simulink model "GolfSwing3D_SimscapePhysicalInterfaceSwitching"  (R2024b)
settings: Solver=VariableStepAuto  StartTime=0.0  StopTime=StopTime  MaxStep=0.001  RelTol=1e-3
model workspace: external: MAT-File 3DModelInputs.mat (data not in the file)
undefined symbols (not defined in the file): GripStrength, KillswitchFinalValue, KillswitchInitialValue, KillswitchStepTime, LeftLowerArmLength, PlaneTilt, RightLowerArmLength, UpperTorsoLength, X, Y, Z
libraries: nesl_utility x363, sm_lib x137, matrix_library x11, fl_lib x8, simulink x1
(part 5 of 13)

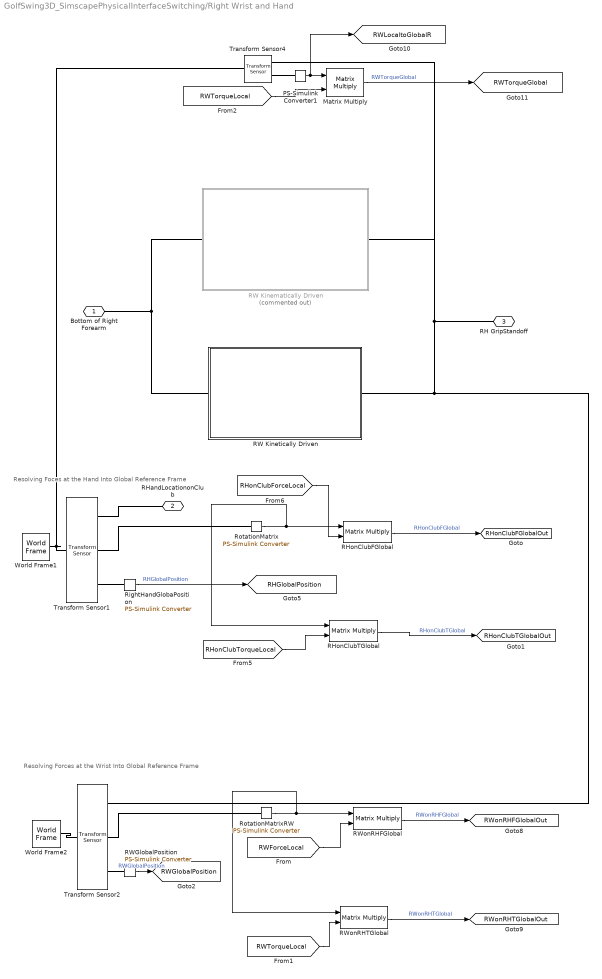
== system GolfSwing3D_SimscapePhysicalInterfaceSwitching/Right Wrist and Hand ==
  note: Resolving Foces at the Hand Into Global Reference Frame
  note: Resolving Forces at the Wrist Into Global Reference Frame
  Matrix Multiply : Product  Multiplication=Matrix(*)
  PS-Simulink Converter1 : nesl_utility/PS-Simulink Converter  PhysicalDomain=network_engine_domain  SubClassName=ps_output  LeftPortType=input  RightPortType=output  PseudoPeriodic=off  Frequencies=[]  VectorFormat=1-D array  Unit=inherit  AffineConversion=off
  RHonClubFGlobal : Product  Multiplication=Matrix(*)
  RHonClubTGlobal : Product  Multiplication=Matrix(*)
  RW Kinematically Driven : Subsystem  Commented=on
  RW Kinetically Driven : Subsystem
  RWGlobalPosition : nesl_utility/PS-Simulink Converter  PhysicalDomain=network_engine_domain  SubClassName=ps_output  LeftPortType=input  RightPortType=output  PseudoPeriodic=off  Frequencies=[]  VectorFormat=1-D array  Unit=inherit  AffineConversion=off
  RWonRHFGlobal : Product  Multiplication=Matrix(*)
  RWonRHTGlobal : Product  Multiplication=Matrix(*)
  RightHandGlobaPosition : nesl_utility/PS-Simulink Converter  PhysicalDomain=network_engine_domain  SubClassName=ps_output  LeftPortType=input  RightPortType=output  PseudoPeriodic=off  Frequencies=[]  VectorFormat=1-D array  Unit=inherit  AffineConversion=off
  RotationMatrix : nesl_utility/PS-Simulink Converter  PhysicalDomain=network_engine_domain  SubClassName=ps_output  LeftPortType=input  RightPortType=output  PseudoPeriodic=off  Frequencies=[]  VectorFormat=1-D array  Unit=inherit  AffineConversion=off
  RotationMatrixRW : nesl_utility/PS-Simulink Converter  PhysicalDomain=network_engine_domain  SubClassName=ps_output  LeftPortType=input  RightPortType=output  PseudoPeriodic=off  Frequencies=[]  VectorFormat=1-D array  Unit=inherit  AffineConversion=off
  Transform Sensor1 : sm_lib/Frames and Transforms/Transform Sensor  MeasurementFrame=World  RotationSequence=XYX  SenseAngle=off  SenseAxis=off  SenseQ=off  SenseR=on  SenseRotationSequence=off  SenseOmegaX=off  SenseOmegaY=off  SenseOmegaZ=off  SenseOmega=off  SenseQDot=off  SenseRDot=off  SenseRotationSequenceDot=off  SenseAlphaX=off  SenseAlphaY=off  SenseAlphaZ=off  SenseAlpha=off  SenseQDDot=off  SenseRDDot=off  SenseX=off  SenseY=off  SenseZ=off  SenseXYZ=on  SenseRad=off  SenseAzim=off  SenseDist=off  SenseInc=off  SenseXDot=off  SenseYDot=off  SenseZDot=off  SenseXYZDot=off  SenseRadDot=off  SenseAzimDot=off  SenseDistDot=off  SenseIncDot=off  SenseXDDot=off  SenseYDDot=off  SenseZDDot=off  SenseXYZDDot=off  SenseRadDDot=off  SenseAzimDDot=off  SenseDistDDot=off  SenseIncDDot=off
  Transform Sensor2 : sm_lib/Frames and Transforms/Transform Sensor  MeasurementFrame=World  RotationSequence=XYX  SenseAngle=off  SenseAxis=off  SenseQ=off  SenseR=on  SenseRotationSequence=off  SenseOmegaX=off  SenseOmegaY=off  SenseOmegaZ=off  SenseOmega=off  SenseQDot=off  SenseRDot=off  SenseRotationSequenceDot=off  SenseAlphaX=off  SenseAlphaY=off  SenseAlphaZ=off  SenseAlpha=off  SenseQDDot=off  SenseRDDot=off  SenseX=off  SenseY=off  SenseZ=off  SenseXYZ=on  SenseRad=off  SenseAzim=off  SenseDist=off  SenseInc=off  SenseXDot=off  SenseYDot=off  SenseZDot=off  SenseXYZDot=off  SenseRadDot=off  SenseAzimDot=off  SenseDistDot=off  SenseIncDot=off  SenseXDDot=off  SenseYDDot=off  SenseZDDot=off  SenseXYZDDot=off  SenseRadDDot=off  SenseAzimDDot=off  SenseDistDDot=off  SenseIncDDot=off
  Transform Sensor4 : sm_lib/Frames and Transforms/Transform Sensor  MeasurementFrame=World  RotationSequence=XYX  SenseAngle=off  SenseAxis=off  SenseQ=off  SenseR=on  SenseRotationSequence=off  SenseOmegaX=off  SenseOmegaY=off  SenseOmegaZ=off  SenseOmega=off  SenseQDot=off  SenseRDot=off  SenseRotationSequenceDot=off  SenseAlphaX=off  SenseAlphaY=off  SenseAlphaZ=off  SenseAlpha=off  SenseQDDot=off  SenseRDDot=off  SenseX=off  SenseY=off  SenseZ=off  SenseXYZ=off  SenseRad=off  SenseAzim=off  SenseDist=off  SenseInc=off  SenseXDot=off  SenseYDot=off  SenseZDot=off  SenseXYZDot=off  SenseRadDot=off  SenseAzimDot=off  SenseDistDot=off  SenseIncDot=off  SenseXDDot=off  SenseYDDot=off  SenseZDDot=off  SenseXYZDDot=off  SenseRadDDot=off  SenseAzimDDot=off  SenseDistDDot=off  SenseIncDDot=off
  World Frame1 : sm_lib/Frames and Transforms/World Frame
  World Frame2 : sm_lib/Frames and Transforms/World Frame
  Bottom of Right Forearm : PMIOPort  Side=Left
  RHandLocationonClub : PMIOPort  Port=2  Side=Right
  RH GripStandoff : PMIOPort  Port=3  Side=Right
  tag scope: RHGlobalPosition=global, RHonClubFGlobalOut=global, RHonClubTGlobalOut=global, RWGlobalPosition=global, RWLocaltoGlobalR=global, RWTorqueGlobal=global, RWonRHFGlobalOut=global, RWonRHTGlobalOut=global
  wires:
  [RHonClubForceLocal] -> RHonClubFGlobal/2
  RotationMatrix/1 -> RHonClubTGlobal/1, RHonClubFGlobal/1
  RHonClubFGlobal/1 -> [RHonClubFGlobalOut]  "RHonClubFGlobal"
  RHonClubTGlobal/1 -> [RHonClubTGlobalOut]  "RHonClubTGlobal"
  [RHonClubTorqueLocal] -> RHonClubTGlobal/2
  RWonRHTGlobal/1 -> [RWonRHTGlobalOut]  "RWonRHTGlobal"
  RotationMatrixRW/1 -> RWonRHTGlobal/1, RWonRHFGlobal/1
  RWGlobalPosition/1 -> [RWGlobalPosition]  "RWGlobalPosition"
  RWonRHFGlobal/1 -> [RWonRHFGlobalOut]  "RWonRHFGlobal"
  RightHandGlobaPosition/1 -> [RHGlobalPosition]  "RHGlobalPosition"
  [RWForceLocal] -> RWonRHFGlobal/2
  [RWTorqueLocal] -> RWonRHTGlobal/2
  PS-Simulink Converter1/1 -> [RWLocaltoGlobalR], Matrix Multiply/1
  Matrix Multiply/1 -> [RWTorqueGlobal]  "RWTorqueGlobal"
  [RWTorqueLocal] -> Matrix Multiply/2
  connections:
  RotationMatrix/LConn1 -- Transform Sensor1/RConn2
  World Frame1/RConn1 -- Transform Sensor4/LConn1 -- Transform Sensor1/LConn1
  Transform Sensor1/RConn3 -- RightHandGlobaPosition/LConn1
  RHandLocationonClub/RConn1 -- Transform Sensor1/RConn1
  RotationMatrixRW/LConn1 -- Transform Sensor2/RConn2
  World Frame2/RConn1 -- Transform Sensor2/LConn1
  Transform Sensor2/RConn3 -- RWGlobalPosition/LConn1
  Transform Sensor2/RConn1 -- Transform Sensor4/RConn1 -- RW Kinematically Driven/RConn1 -- RH GripStandoff/RConn1 -- RW Kinetically Driven/RConn1
  RW Kinetically Driven/LConn1 -- RW Kinematically Driven/LConn1 -- Bottom of Right Forearm/RConn1
  Transform Sensor4/RConn2 -- PS-Simulink Converter1/LConn1

== system GolfSwing3D_SimscapePhysicalInterfaceSwitching/Spine Input Function ==
  Spine Bending Torques : MATLAB Function  TreatAsAtomicUnit=on  SystemSampleTime=0
  tag scope: FcnOutSpineAccelerationX=global, FcnOutSpineAccelerationY=global, FcnOutSpinePositionX=global, FcnOutSpinePositionY=global, FcnOutSpineTorqueX=global, FcnOutSpineTorqueY=global, FcnOutSpineVelocityX=global, FcnOutSpineVelocityY=global
  wires:
  Spine Bending Torques/2(JointTorqueSpineY) -> [FcnOutSpineTorqueY]  "SpineTorqueYInput"
  [Time] -> Spine Bending Torques/1(Time)
  Spine Bending Torques/1(JointTorqueSpineX) -> [FcnOutSpineTorqueX]  "SpineTorqueXInput"
  [Killswitch] -> Spine Bending Torques/2(Killswitch)
  [SpineVelocityY] -> Spine Bending Torques/6(SpineVelocityY)
  [SpineVelocityX] -> Spine Bending Torques/5(SpineVelocityX)
  [SpinePositionY] -> Spine Bending Torques/4(SpinePositionY)
  [SpinePositionX] -> Spine Bending Torques/3(SpinePositionX)
  Spine Bending Torques/3(SpinePositionInputX) -> [FcnOutSpinePositionX]
  Spine Bending Torques/4(SpinePositionInputY) -> [FcnOutSpinePositionY]
  Spine Bending Torques/5(SpineVelocityInputX) -> [FcnOutSpineVelocityX]
  Spine Bending Torques/6(SpineVelocityInputY) -> [FcnOutSpineVelocityY]
  Spine Bending Torques/7(SpineAccelerationInputX) -> [FcnOutSpineAccelerationX]
  Spine Bending Torques/8(SpineAccelerationInputY) -> [FcnOutSpineAccelerationY]

== system GolfSwing3D_SimscapePhysicalInterfaceSwitching/Torso Input Function ==
  Torso Input Torque : MATLAB Function  TreatAsAtomicUnit=on  SystemSampleTime=0
  tag scope: FcnOutTorsoAcceleration=global, FcnOutTorsoPosition=global, FcnOutTorsoTorque=global, FcnOutTorsoVelocity=global
  wires:
  [TorsoPosition] -> Torso Input Torque/3(TorsoPosition)  "TorsoPositionIn"
  Torso Input Torque/4(TorsoAccelerationInput) -> [FcnOutTorsoAcceleration]  "FcnOutTorsoAcceleration"
  [TorsoVelocity] -> Torso Input Torque/4(TorsoVelocity)  "TorsoVelocityIn"
  Torso Input Torque/1(JointTorqueTorso) -> [FcnOutTorsoTorque]  "TorsoTorqueInput"
  [Killswitch] -> Torso Input Torque/2(Killswitch)
  Torso Input Torque/2(TorsoPositionInput) -> [FcnOutTorsoPosition]  "FcnOutTorsoPosition"
  Torso Input Torque/3(TorsoVelocityInput) -> [FcnOutTorsoVelocity]  "FcnOutTorsoVelocity"
  [Time] -> Torso Input Torque/1(Time)

== system GolfSwing3D_SimscapePhysicalInterfaceSwitching/Translation Input Function ==
  ConvertGlobalXtoHipBaseLocal : Product  Multiplication=Matrix(*)
  Demux : Demux  Outputs=3
  GlobalBaseTranslationalForce : MATLAB Function  TreatAsAtomicUnit=on  SystemSampleTime=0
  Mux : Mux  Inputs=3
  tag scope: FcnOutTranslationAccelerationX=global, FcnOutTranslationAccelerationY=global, FcnOutTranslationAccelerationZ=global, FcnOutTranslationForceX=global, FcnOutTranslationForceY=global, FcnOutTranslationForceZ=global, FcnOutTranslationPositionX=global, FcnOutTranslationPositionY=global, FcnOutTranslationPositionZ=global, FcnOutTranslationVelocityX=global, FcnOutTranslationVelocityY=global, FcnOutTranslationVelocityZ=global
  wires:
  Mux/1 -> ConvertGlobalXtoHipBaseLocal/2
  [Killswitch] -> GlobalBaseTranslationalForce/2(Killswitch)
  ConvertGlobalXtoHipBaseLocal/1 -> Demux/1  "BaseonHipForceHipBase"
  GlobalBaseTranslationalForce/8(TranslationVelocityInputY) -> [FcnOutTranslationVelocityY]
  GlobalBaseTranslationalForce/3(TranslationForceZ) -> Mux/3  "TranslationForceZInput"
  GlobalBaseTranslationalForce/1(TranslationForceX) -> Mux/1  "TranslationForceXInput"
  GlobalBaseTranslationalForce/11(TranslationAccelerationInputY) -> [FcnOutTranslationAccelerationY]
  Demux/3 -> [FcnOutTranslationForceZ]  "BaseonHipForceHipBaseZ"
  GlobalBaseTranslationalForce/2(TranslationForceY) -> Mux/2  "TranslationForceYInput"
  GlobalBaseTranslationalForce/5(TranslationPositionInputY) -> [FcnOutTranslationPositionY]
  GlobalBaseTranslationalForce/4(TranslationPositionInputX) -> [FcnOutTranslationPositionX]
  GlobalBaseTranslationalForce/10(TranslationAccelerationInputX) -> [FcnOutTranslationAccelerationX]
  Demux/2 -> [FcnOutTranslationForceY]  "BaseonHipForceHipBaseY"
  GlobalBaseTranslationalForce/12(TranslationAccelerationInputZ) -> [FcnOutTranslationAccelerationZ]
  [RotationMatrixGlobaltoHipJointBase] -> ConvertGlobalXtoHipBaseLocal/1
  GlobalBaseTranslationalForce/9(TranslationVelocityInputZ) -> [FcnOutTranslationVelocityZ]
  [Time] -> GlobalBaseTranslationalForce/1(Time)
  Demux/1 -> [FcnOutTranslationForceX]  "BaseonHipForceHipBaseX"
  GlobalBaseTranslationalForce/7(TranslationVelocityInputX) -> [FcnOutTranslationVelocityX]
  GlobalBaseTranslationalForce/6(TranslationPositionInputZ) -> [FcnOutTranslationPositionZ]
  [HipGlobalPositionX] -> GlobalBaseTranslationalForce/3(TranslationPositionX)
  [HipGlobalPositionY] -> GlobalBaseTranslationalForce/4(TranslationPositionY)
  [HipGlobalPositionZ] -> GlobalBaseTranslationalForce/5(TranslationPositionZ)
  [HipGlobalVelocityX] -> GlobalBaseTranslationalForce/6(TranslationVelocityX)
  [HipGlobalVelocityY] -> GlobalBaseTranslationalForce/7(TranslationVelocityY)
  [HipGlobalVelocityZ] -> GlobalBaseTranslationalForce/8(TranslationVelocityZ)

== system GolfSwing3D_SimscapePhysicalInterfaceSwitching/Club/Flexible Beam Model ==
  Flexible Cylindrical Beam : sm_lib/Body Elements/Flexible Bodies/Beams/Flexible Cylindrical Beam  SectionType=Hollow  Radius=0.010  RadiusUnits=m  Thickness=0.0015  ThicknessUnits=m  Length=ShaftLength  LengthUnits=m  StiffnessAndInertiaType=CalculateFromGeometry  Density=500  DensityUnits=kg/m^3  ModuliType=YoungsPoissons  YoungsModulus=ShaftStiffness  YoungsModulusUnits=GPa  PoissonsRatio=0.33  ShearModulus=26  ShearModulusUnits=GPa  GeometricCentroid=[0 0]  GeometricCentroidUnits=m  BendingCentroid=[0 0]  BendingCentroidUnits=m  ShearCenter=[0 0]  ShearCenterUnits=m  AxialRigidity=1  AxialRigidityUnits=Pa*m^2  FlexuralRigidity=[1 1]  FlexuralRigidityUnits=Pa*m^4  CrossFlexuralRigidity=0  CrossFlexuralRigidityUnits=Pa*m^4  TorsionalRigidity=1  TorsionalRigidityUnits=Pa*m^4  CenterOfMass=[0 0]  CenterOfMassUnits=m  MassPerUnitLength=1  MassPerUnitLengthUnits=kg/m  MassMomentOfInertiaDensity=[1 1]  MassMomentOfInertiaDensityUnits=kg*m  MassProductOfInertiaDensity=0  MassProductOfInertiaDensityUnits=kg*m  DampingType=Proportional  ProportionalDampingAlpha=0  ProportionalDampingAlphaUnits=1/s  ProportionalDampingBeta=ShaftDampening  ProportionalDampingBetaUnits=s  UniformModalDampingRatio=0.01  NumElements=2  ReductionType=None  NumRetainedModes=1  GraphicType=FromGeometry  GraphicVisPropType=SimpleVisualProperties  GraphicDiffuseColor=[0.5 0.5 0.5]  GraphicOpacity=1.0  GraphicSpecularColor=[0.5 0.5 0.5 1.0]  GraphicAmbientColor=[0.15 0.15 0.15 1.0]  GraphicEmissiveColor=[0.0 0.0 0.0 1.0]  GraphicShininess=75  DoExposeZminFrame=on  DoExposeZmaxFrame=on  SerializedFrames=<Frames/>
  Rigid Transform : sm_lib/Frames and Transforms/Rigid Transform  RotationMethod=RotationSequence  FollAlignAxisA=+X  BaseAlignAxisA=+Y  FollAlignAxisB=+Y  BaseAlignAxisB=+Z  RotationStandardAxis=+Z  RotationAngle=0.0  RotationAngleUnits=deg  RotationArbitraryAxis=[0 0 1]  RotationSequenceAxes=FollowerAxes  RotationSequence=XYX  RotationSequenceAngles=[0 90 0]  RotationSequenceAnglesUnits=deg  RotationMatrix=[1 0 0; 0 1 0; 0 0 1]  Quaternion=[1 0 0 0]  TranslationMethod=None  TranslationCartesianOffset=[0 0 0]  TranslationCartesianOffsetUnits=m  TranslationStandardAxis=+Z  TranslationStandardOffset=0  TranslationStandardOffsetUnits=m  TranslationROffset=0  TranslationROffsetUnits=m  TranslationThetaOffset=0  TranslationThetaOffsetUnits=deg  TranslationZOffset=0  TranslationZOffsetUnits=m
  RH Grip : PMIOPort  Side=Left
  Clubhead : PMIOPort  Port=2  Side=Right
  connections:
  Rigid Transform/RConn1 -- Flexible Cylindrical Beam/LConn1
  RH Grip/RConn1 -- Rigid Transform/LConn1
  Flexible Cylindrical Beam/RConn1 -- Clubhead/RConn1

== system GolfSwing3D_SimscapePhysicalInterfaceSwitching/Club/Rigid Shaft ==
  Rigid Shaft : sm_lib/Body Elements/Cylindrical Solid  CylinderRadius=0.01  CylinderRadiusUnits=m  CylinderLength=1  CylinderLengthUnits=m  ExportEntireGeometry=off  InertiaType=CalculateFromGeometry  BasedOnType=Mass  Density=500  DensityUnits=kg/m^3  Mass=0.0802566  MassUnits=kg  CenterOfMass=[0 0 0]  CenterOfMassUnits=m  MomentsOfInertia=[1 1 1]  MomentsOfInertiaUnits=kg*m^2  ProductsOfInertia=[0 0 0]  ProductsOfInertiaUnits=kg*m^2  GraphicType=FromGeometry  MarkerShape=Sphere  MarkerSize=10  GraphicVisPropType=SimpleVisualProperties  GraphicDiffuseColor=[0.5 0.5 0.5]  GraphicOpacity=1.0  GraphicSpecularColor=[0.5 0.5 0.5 1.0]  GraphicAmbientColor=[0.15 0.15 0.15 1.0]  GraphicEmissiveColor=[0.0 0.0 0.0 1.0]  GraphicShininess=75  DoExposeReferenceFrame=off  SerializedFrames=<Frames><Frame><Id>Frame1</Id><Value><Name>RHGripTOS</Name><Origin><Source>GeometricFeature</Source><FeatureName>top curve</FeatureName></Origin><PrimaryAxis><DefinedDirection>-X</DefinedDirection><Source>ReferenceFrame</Source><SourceDirection>+Z</SourceDirection><FeatureName></FeatureName></PrimaryAxis><SecondaryAxis><DefinedDirection>+Y</DefinedDirection><Source>ReferenceFrame</Source><SourceDirection>+X</SourceDirection><FeatureName></FeatureName></SecondaryAxis></Value></Frame><Frame><Id>Frame2</Id><Value><Name>ShaftS1</Name><Origin><Source>GeometricFeature</Source><FeatureName>bottom curve</FeatureName></Origin><PrimaryAxis><DefinedDirection>-X</DefinedDirection><Source>ReferenceFrame</Source><SourceDirection>+Z</SourceDirection><FeatureName></FeatureName></PrimaryAxis><SecondaryAxis><DefinedDirection>+Y</DefinedDirection><Source>ReferenceFrame</Source><SourceDirection>+X</SourceDirection><FeatureName></FeatureName></SecondaryAxis></Value></Frame></Frames>
  RH : PMIOPort  Side=Right
  Clubhead : PMIOPort  Port=2  Side=Right
  connections:
  RH/RConn1 -- Rigid Shaft/LConn1
  Clubhead/RConn1 -- Rigid Shaft/RConn1

== system GolfSwing3D_SimscapePhysicalInterfaceSwitching/Club/Zero Mass Reference Shaft ==
  CHSCalculation : Subsystem  Commented=on
  CHvx : nesl_utility/PS-Simulink Converter  Commented=on  PhysicalDomain=network_engine_domain  SubClassName=ps_output  LeftPortType=input  RightPortType=output  PseudoPeriodic=off  Frequencies=[]  VectorFormat=1-D array  Unit=inherit  AffineConversion=off
  CHvy : nesl_utility/PS-Simulink Converter  Commented=on  PhysicalDomain=network_engine_domain  SubClassName=ps_output  LeftPortType=input  RightPortType=output  PseudoPeriodic=off  Frequencies=[]  VectorFormat=1-D array  Unit=inherit  AffineConversion=off
  CHvz : nesl_utility/PS-Simulink Converter  Commented=on  PhysicalDomain=network_engine_domain  SubClassName=ps_output  LeftPortType=input  RightPortType=output  PseudoPeriodic=off  Frequencies=[]  VectorFormat=1-D array  Unit=inherit  AffineConversion=off
  CHx : nesl_utility/PS-Simulink Converter  Commented=on  PhysicalDomain=network_engine_domain  SubClassName=ps_output  LeftPortType=input  RightPortType=output  PseudoPeriodic=off  Frequencies=[]  VectorFormat=1-D array  Unit=inherit  AffineConversion=off
  CHy : nesl_utility/PS-Simulink Converter  Commented=on  PhysicalDomain=network_engine_domain  SubClassName=ps_output  LeftPortType=input  RightPortType=output  PseudoPeriodic=off  Frequencies=[]  VectorFormat=1-D array  Unit=inherit  AffineConversion=off
  CHz : nesl_utility/PS-Simulink Converter  Commented=on  PhysicalDomain=network_engine_domain  SubClassName=ps_output  LeftPortType=input  RightPortType=output  PseudoPeriodic=off  Frequencies=[]  VectorFormat=1-D array  Unit=inherit  AffineConversion=off
  ClubheadPathUnitVector : Mux  Commented=on  Inputs=3
  ShaftPhysicalConfig : Subsystem
  Transform Sensor : sm_lib/Frames and Transforms/Transform Sensor  Commented=on  MeasurementFrame=World  RotationSequence=XYX  SenseAngle=off  SenseAxis=off  SenseQ=off  SenseR=off  SenseRotationSequence=off  SenseOmegaX=off  SenseOmegaY=off  SenseOmegaZ=off  SenseOmega=off  SenseQDot=off  SenseRDot=off  SenseRotationSequenceDot=off  SenseAlphaX=off  SenseAlphaY=off  SenseAlphaZ=off  SenseAlpha=off  SenseQDDot=off  SenseRDDot=off  SenseX=on  SenseY=on  SenseZ=on  SenseXYZ=off  SenseRad=off  SenseAzim=off  SenseDist=off  SenseInc=off  SenseXDot=on  SenseYDot=on  SenseZDot=on  SenseXYZDot=off  SenseRadDot=off  SenseAzimDot=off  SenseDistDot=off  SenseIncDot=off  SenseXDDot=off  SenseYDDot=off  SenseZDDot=off  SenseXYZDDot=off  SenseRadDDot=off  SenseAzimDDot=off  SenseDistDDot=off  SenseIncDDot=off
  UnitVectorX : Product  Commented=on  Inputs=*/
  UnitVectorY : Product  Commented=on  Inputs=*/
  UnitVectorZ : Product  Commented=on  Inputs=*/
  RH : PMIOPort  Side=Right
  ConnGlobal : PMIOPort  Port=2  Side=Right
  wires:
  CHvz/1 -> CHSCalculation/3(In1), UnitVectorZ/1
  CHvy/1 -> CHSCalculation/2(In3), UnitVectorY/1
  UnitVectorY/1 -> ClubheadPathUnitVector/2
  UnitVectorZ/1 -> ClubheadPathUnitVector/3
  CHSCalculation/1(Out1) -> UnitVectorY/2, UnitVectorZ/2, UnitVectorX/2  "GhostCHS"
  UnitVectorX/1 -> ClubheadPathUnitVector/1
  CHvx/1 -> CHSCalculation/1(In2), UnitVectorX/1
  connections:
  ShaftPhysicalConfig/RConn1 -- RH/RConn1
  ConnGlobal/RConn1 -- Transform Sensor/LConn1
  ShaftPhysicalConfig/RConn2 -- Transform Sensor/RConn1
  CHy/LConn1 -- Transform Sensor/RConn3
  CHvy/LConn1 -- Transform Sensor/RConn6
  CHx/LConn1 -- Transform Sensor/RConn2
  CHz/LConn1 -- Transform Sensor/RConn4
  CHvz/LConn1 -- Transform Sensor/RConn7
  CHvx/LConn1 -- Transform Sensor/RConn5

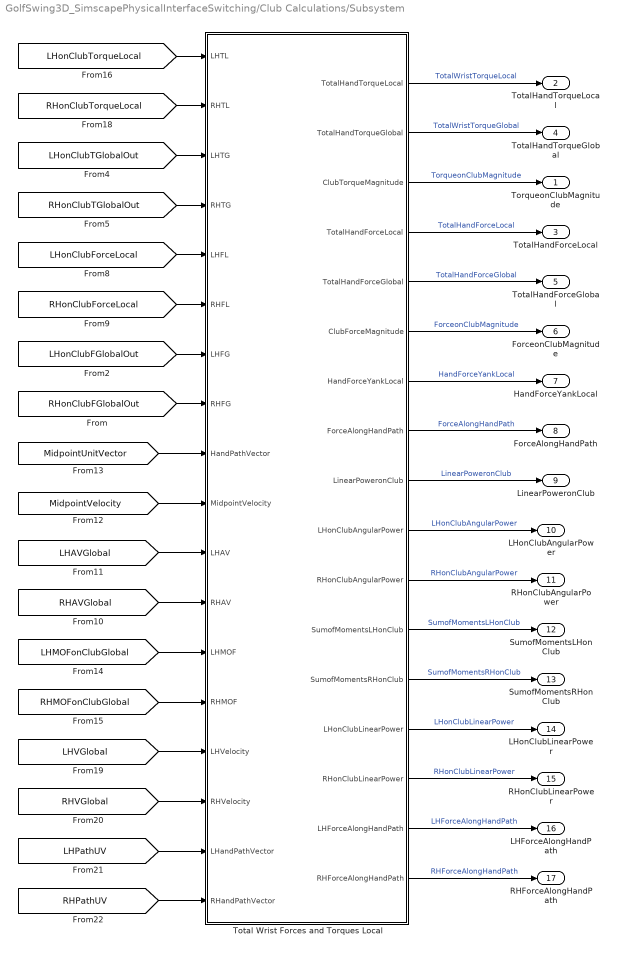
== system GolfSwing3D_SimscapePhysicalInterfaceSwitching/Club Calculations/Subsystem ==
  Total Wrist Forces and Torques Local : MATLAB Function  TreatAsAtomicUnit=on  SystemSampleTime=0
  TorqueonClubMagnitude : Outport  PortDimensions=1
  TotalHandTorqueLocal : Outport  Port=2  PortDimensions=3
  TotalHandForceLocal : Outport  Port=3  PortDimensions=3
  TotalHandTorqueGlobal : Outport  Port=4  PortDimensions=3
  TotalHandForceGlobal : Outport  Port=5  PortDimensions=3
  ForceonClubMagnitude : Outport  Port=6  PortDimensions=1
  HandForceYankLocal : Outport  Port=7  PortDimensions=2
  ForceAlongHandPath : Outport  Port=8  PortDimensions=1
  LinearPoweronClub : Outport  Port=9  PortDimensions=1
  LHonClubAngularPower : Outport  Port=10  PortDimensions=1
  RHonClubAngularPower : Outport  Port=11  PortDimensions=1
  SumofMomentsLHonClub : Outport  Port=12  PortDimensions=3
  SumofMomentsRHonClub : Outport  Port=13  PortDimensions=3
  LHonClubLinearPower : Outport  Port=14  PortDimensions=1
  RHonClubLinearPower : Outport  Port=15
  LHForceAlongHandPath : Outport  Port=16  PortDimensions=1
  RHForceAlongHandPath : Outport  Port=17  PortDimensions=1
  wires:
  [LHonClubTGlobalOut] -> Total Wrist Forces and Torques Local/3(LHTG)
  [MidpointUnitVector] -> Total Wrist Forces and Torques Local/9(HandPathVector)
  [RHonClubForceLocal] -> Total Wrist Forces and Torques Local/6(RHFL)
  [RHonClubTorqueLocal] -> Total Wrist Forces and Torques Local/2(RHTL)
  [LHonClubFGlobalOut] -> Total Wrist Forces and Torques Local/7(LHFG)
  [LHonClubForceLocal] -> Total Wrist Forces and Torques Local/5(LHFL)
  [RHAVGlobal] -> Total Wrist Forces and Torques Local/12(RHAV)
  [LHPathUV] -> Total Wrist Forces and Torques Local/17(LHandPathVector)
  [RHonClubTGlobalOut] -> Total Wrist Forces and Torques Local/4(RHTG)
  [MidpointVelocity] -> Total Wrist Forces and Torques Local/10(MidpointVelocity)
  [LHVGlobal] -> Total Wrist Forces and Torques Local/15(LHVelocity)
  [RHVGlobal] -> Total Wrist Forces and Torques Local/16(RHVelocity)
  [RHonClubFGlobalOut] -> Total Wrist Forces and Torques Local/8(RHFG)
  Total Wrist Forces and Torques Local/15(RHonClubLinearPower) -> RHonClubLinearPower/1  "RHonClubLinearPower"
  Total Wrist Forces and Torques Local/4(TotalHandForceLocal) -> TotalHandForceLocal/1  "TotalHandForceLocal"
  [RHPathUV] -> Total Wrist Forces and Torques Local/18(RHandPathVector)
  [LHMOFonClubGlobal] -> Total Wrist Forces and Torques Local/13(LHMOF)
  [LHAVGlobal] -> Total Wrist Forces and Torques Local/11(LHAV)
  Total Wrist Forces and Torques Local/5(TotalHandForceGlobal) -> TotalHandForceGlobal/1  "TotalHandForceGlobal"
  [LHonClubTorqueLocal] -> Total Wrist Forces and Torques Local/1(LHTL)
  Total Wrist Forces and Torques Local/6(ClubForceMagnitude) -> ForceonClubMagnitude/1  "ForceonClubMagnitude"
  Total Wrist Forces and Torques Local/7(HandForceYankLocal) -> HandForceYankLocal/1  "HandForceYankLocal"
  [RHMOFonClubGlobal] -> Total Wrist Forces and Torques Local/14(RHMOF)
  Total Wrist Forces and Torques Local/13(SumofMomentsRHonClub) -> SumofMomentsRHonClub/1  "SumofMomentsRHonClub"
  Total Wrist Forces and Torques Local/16(LHForceAlongHandPath) -> LHForceAlongHandPath/1  "LHForceAlongHandPath"
  Total Wrist Forces and Torques Local/12(SumofMomentsLHonClub) -> SumofMomentsLHonClub/1  "SumofMomentsLHonClub"
  Total Wrist Forces and Torques Local/9(LinearPoweronClub) -> LinearPoweronClub/1  "LinearPoweronClub"
  Total Wrist Forces and Torques Local/8(ForceAlongHandPath) -> ForceAlongHandPath/1  "ForceAlongHandPath"
  Total Wrist Forces and Torques Local/14(LHonClubLinearPower) -> LHonClubLinearPower/1  "LHonClubLinearPower"
  Total Wrist Forces and Torques Local/11(RHonClubAngularPower) -> RHonClubAngularPower/1  "RHonClubAngularPower"
  Total Wrist Forces and Torques Local/3(ClubTorqueMagnitude) -> TorqueonClubMagnitude/1  "TorqueonClubMagnitude"
  Total Wrist Forces and Torques Local/10(LHonClubAngularPower) -> LHonClubAngularPower/1  "LHonClubAngularPower"
  Total Wrist Forces and Torques Local/2(TotalHandTorqueGlobal) -> TotalHandTorqueGlobal/1  "TotalWristTorqueGlobal"
  Total Wrist Forces and Torques Local/1(TotalHandTorqueLocal) -> TotalHandTorqueLocal/1  "TotalWristTorqueLocal"
  Total Wrist Forces and Torques Local/17(RHForceAlongHandPath) -> RHForceAlongHandPath/1  "RHForceAlongHandPath"

== system GolfSwing3D_SimscapePhysicalInterfaceSwitching/Club Calculations/Work and Impulse Integrators ==
  LHLinearWorkonClub : Integrator
  LWAngularImpulseonClub : Integrator
  LWAngularWorkonClub : Integrator
  LeftHandLinearImpulse : Integrator
  LinearImpulseonClub : Integrator
  LinearWorkonClub : Integrator
  RHLinearWorkOnClub : Integrator
  RWAngularImpulseonClub : Integrator
  RWAngularWorkonClub : Integrator
  RightHandLinearImpulseonClub : Integrator
  wires:
  [TotalHandForceGlobal] -> LinearImpulseonClub/1
  [LHonClubLinearPower] -> LHLinearWorkonClub/1
  [LinearPoweronClub] -> LinearWorkonClub/1
  [RHonClubAngularPower] -> RWAngularWorkonClub/1
  [RHonClubFGlobalOut] -> RightHandLinearImpulseonClub/1
  [LHonClubFGlobalOut] -> LeftHandLinearImpulse/1
  [LHonClubAngularPower] -> LWAngularWorkonClub/1
  [SumofMomentsRHonClub] -> RWAngularImpulseonClub/1
  [SumofMomentsLHonClub] -> LWAngularImpulseonClub/1
  [RHonClubLinearPower] -> RHLinearWorkOnClub/1

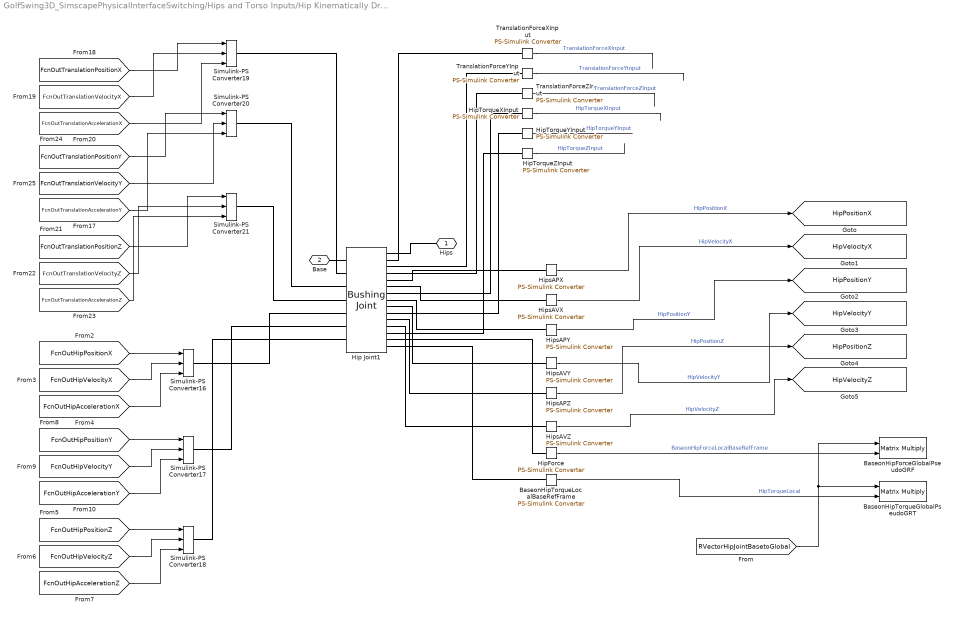
== system GolfSwing3D_SimscapePhysicalInterfaceSwitching/Hips and Torso Inputs/Hip Kinematically Driven ==
  BaseonHipForceGlobalPseudoGRF : Product  Multiplication=Matrix(*)
  BaseonHipTorqueGlobalPseudoGRT : Product  Multiplication=Matrix(*)
  BaseonHipTorqueLocalBaseRefFrame : nesl_utility/PS-Simulink Converter  PhysicalDomain=network_engine_domain  SubClassName=ps_output  LeftPortType=input  RightPortType=output  PseudoPeriodic=off  Frequencies=[]  VectorFormat=1-D array  Unit=inherit  AffineConversion=off
  Hip Joint1 : sm_lib/Joints/Bushing Joint  JointMode=Normal  CompositeWrenchDir=BaseOnFollower  CompositeWrenchFrame=BaseFrame  SenseConstraintForce=off  SenseConstraintTorque=off  SenseTotalForce=on  SenseTotalTorque=on  PxPositionTargetSpecify=off  PxPositionTargetPriority=High  PxPositionTargetValue=TranslationStartPositionX  PxPositionTargetValueUnits=m  PxVelocityTargetSpecify=off  PxVelocityTargetPriority=High  PxVelocityTargetValue=TranslationStartVelocityX  PxVelocityTargetValueUnits=m/s  PxEquilibriumPosition=0  PxEquilibriumPositionUnits=m  PxSpringStiffness=0  PxSpringStiffnessUnits=N/m  PxDampingCoefficient=0  PxDampingCoefficientUnits=N/(m/s)  PxLowerLimitSpecify=off  PxLowerLimitBound=-1  PxLowerLimitBoundUnits=m  PxLowerLimitStiffness=1e6  PxLowerLimitStiffnessUnits=N/m  PxLowerLimitDamping=1e3  PxLowerLimitDampingUnits=N/(m/s)  PxLowerLimitTransitionRegionWidth=1e-4  PxLowerLimitTransitionRegionWidthUnits=m  PxUpperLimitSpecify=off  PxUpperLimitBound=1  PxUpperLimitBoundUnits=m  PxUpperLimitStiffness=1e6  PxUpperLimitStiffnessUnits=N/m  PxUpperLimitDamping=1e3  PxUpperLimitDampingUnits=N/(m/s)  PxUpperLimitTransitionRegionWidth=1e-4  PxUpperLimitTransitionRegionWidthUnits=m  PxTorqueActuationMode=ComputedTorque  PxMotionActuationMode=InputMotion  PxSensePosition=off  PxSenseVelocity=off  PxSenseAcceleration=off  PxSenseTorqueForce=on  PxSenseLowerLimitTorqueForce=off  PxSenseUpperLimitTorqueForce=off  PyPositionTargetSpecify=off  PyPositionTargetPriority=High  PyPositionTargetValue=TranslationStartPositionY  PyPositionTargetValueUnits=m  PyVelocityTargetSpecify=off  PyVelocityTargetPriority=High  PyVelocityTargetValue=TranslationStartVelocityY  PyVelocityTargetValueUnits=m/s  PyEquilibriumPosition=0  PyEquilibriumPositionUnits=m  PySpringStiffness=0  PySpringStiffnessUnits=N/m  PyDampingCoefficient=0  PyDampingCoefficientUnits=N/(m/s)  PyLowerLimitSpecify=off  PyLowerLimitBound=-1  PyLowerLimitBoundUnits=m  PyLowerLimitStiffness=1e6  PyLowerLimitStiffnessUnits=N/m  PyLowerLimitDamping=1e3  PyLowerLimitDampingUnits=N/(m/s)  PyLowerLimitTransitionRegionWidth=1e-4  PyLowerLimitTransitionRegionWidthUnits=m  PyUpperLimitSpecify=off  PyUpperLimitBound=1  PyUpperLimitBoundUnits=m  PyUpperLimitStiffness=1e6  PyUpperLimitStiffnessUnits=N/m  PyUpperLimitDamping=1e3  PyUpperLimitDampingUnits=N/(m/s)  PyUpperLimitTransitionRegionWidth=1e-4  PyUpperLimitTransitionRegionWidthUnits=m  PyTorqueActuationMode=ComputedTorque  PyMotionActuationMode=InputMotion  PySensePosition=off  PySenseVelocity=off  PySenseAcceleration=off  PySenseTorqueForce=on  PySenseLowerLimitTorqueForce=off  PySenseUpperLimitTorqueForce=off  PzPositionTargetSpecify=off  PzPositionTargetPriority=High  PzPositionTargetValue=TranslationStartPositionZ  PzPositionTargetValueUnits=m  PzVelocityTargetSpecify=off  PzVelocityTargetPriority=High  PzVelocityTargetValue=TranslationStartVelocityZ  PzVelocityTargetValueUnits=m/s  PzEquilibriumPosition=0  PzEquilibriumPositionUnits=m  PzSpringStiffness=0  PzSpringStiffnessUnits=N/m  PzDampingCoefficient=0  PzDampingCoefficientUnits=N/(m/s)  PzLowerLimitSpecify=off  PzLowerLimitBound=-1  PzLowerLimitBoundUnits=m  PzLowerLimitStiffness=1e6  PzLowerLimitStiffnessUnits=N/m  PzLowerLimitDamping=1e3  PzLowerLimitDampingUnits=N/(m/s)  PzLowerLimitTransitionRegionWidth=1e-4  PzLowerLimitTransitionRegionWidthUnits=m  PzUpperLimitSpecify=off  PzUpperLimitBound=1  PzUpperLimitBoundUnits=m  PzUpperLimitStiffness=1e6  PzUpperLimitStiffnessUnits=N/m  PzUpperLimitDamping=1e3  PzUpperLimitDampingUnits=N/(m/s)  PzUpperLimitTransitionRegionWidth=1e-4  PzUpperLimitTransitionRegionWidthUnits=m  PzTorqueActuationMode=ComputedTorque  PzMotionActuationMode=InputMotion  PzSensePosition=off  PzSenseVelocity=off  PzSenseAcceleration=off  PzSenseTorqueForce=on  PzSenseLowerLimitTorqueForce=off  PzSenseUpperLimitTorqueForce=off  RxPositionTargetSpecify=off  RxPositionTargetPriority=High  RxPositionTargetValue=HipStartPositionX  RxPositionTargetValueUnits=deg  RxVelocityTargetSpecify=off  RxVelocityTargetPriority=High  RxVelocityTargetValue=HipStartVelocityX  RxVelocityTargetValueUnits=deg/s  RxEquilibriumPosition=0  RxEquilibriumPositionUnits=deg  RxSpringStiffness=0  RxSpringStiffnessUnits=N*m/deg  RxDampingCoefficient=0  RxDampingCoefficientUnits=N*m/(deg/s)  RxLowerLimitSpecify=off  RxLowerLimitBound=-90  RxLowerLimitBoundUnits=deg  RxLowerLimitStiffness=1e4  RxLowerLimitStiffnessUnits=N*m/deg  RxLowerLimitDamping=10  RxLowerLimitDampingUnits=N*m/(deg/s)  RxLowerLimitTransitionRegionWidth=0.1  RxLowerLimitTransitionRegionWidthUnits=deg  RxUpperLimitSpecify=off  RxUpperLimitBound=90  RxUpperLimitBoundUnits=deg  RxUpperLimitStiffness=1e4  RxUpperLimitStiffnessUnits=N*m/deg  RxUpperLimitDamping=10  RxUpperLimitDampingUnits=N*m/(deg/s)  RxUpperLimitTransitionRegionWidth=0.1  RxUpperLimitTransitionRegionWidthUnits=deg  RxTorqueActuationMode=ComputedTorque  RxMotionActuationMode=InputMotion  RxSensePosition=on  RxSenseVelocity=on  RxSenseAcceleration=off  RxSenseTorqueForce=on  RxSenseLowerLimitTorqueForce=off  RxSenseUpperLimitTorqueForce=off  RyPositionTargetSpecify=off  RyPositionTargetPriority=High  RyPositionTargetValue=HipStartPositionY  RyPositionTargetValueUnits=deg  RyVelocityTargetSpecify=off  RyVelocityTargetPriority=High  RyVelocityTargetValue=HipStartVelocityY  RyVelocityTargetValueUnits=deg/s  RyEquilibriumPosition=0  RyEquilibriumPositionUnits=deg  RySpringStiffness=0  RySpringStiffnessUnits=N*m/deg  RyDampingCoefficient=0  RyDampingCoefficientUnits=N*m/(deg/s)  RyLowerLimitSpecify=off  RyLowerLimitBound=-90  RyLowerLimitBoundUnits=deg  RyLowerLimitStiffness=1e4  RyLowerLimitStiffnessUnits=N*m/deg  RyLowerLimitDamping=10  RyLowerLimitDampingUnits=N*m/(deg/s)  RyLowerLimitTransitionRegionWidth=0.1  RyLowerLimitTransitionRegionWidthUnits=deg  RyUpperLimitSpecify=off  RyUpperLimitBound=90  RyUpperLimitBoundUnits=deg  RyUpperLimitStiffness=1e4  RyUpperLimitStiffnessUnits=N*m/deg  RyUpperLimitDamping=10  RyUpperLimitDampingUnits=N*m/(deg/s)  RyUpperLimitTransitionRegionWidth=0.1  RyUpperLimitTransitionRegionWidthUnits=deg  RyTorqueActuationMode=ComputedTorque  RyMotionActuationMode=InputMotion  RySensePosition=on  RySenseVelocity=on  RySenseAcceleration=off  RySenseTorqueForce=on  RySenseLowerLimitTorqueForce=off  RySenseUpperLimitTorqueForce=off  RzPositionTargetSpecify=off  RzPositionTargetPriority=High  RzPositionTargetValue=HipStartPositionZ  RzPositionTargetValueUnits=deg  RzVelocityTargetSpecify=off  RzVelocityTargetPriority=High  RzVelocityTargetValue=HipStartVelocityZ  RzVelocityTargetValueUnits=deg/s  RzEquilibriumPosition=0  RzEquilibriumPositionUnits=deg  RzSpringStiffness=0  RzSpringStiffnessUnits=N*m/deg  RzDampingCoefficient=0  RzDampingCoefficientUnits=N*m/(deg/s)  RzLowerLimitSpecify=off  RzLowerLimitBound=-90  RzLowerLimitBoundUnits=deg  RzLowerLimitStiffness=1e4  RzLowerLimitStiffnessUnits=N*m/deg  RzLowerLimitDamping=10  RzLowerLimitDampingUnits=N*m/(deg/s)  RzLowerLimitTransitionRegionWidth=0.1  RzLowerLimitTransitionRegionWidthUnits=deg  RzUpperLimitSpecify=off  RzUpperLimitBound=90  RzUpperLimitBoundUnits=deg  RzUpperLimitStiffness=1e4  RzUpperLimitStiffnessUnits=N*m/deg  RzUpperLimitDamping=10  RzUpperLimitDampingUnits=N*m/(deg/s)  RzUpperLimitTransitionRegionWidth=0.1  RzUpperLimitTransitionRegionWidthUnits=deg  RzTorqueActuationMode=ComputedTorque  RzMotionActuationMode=InputMotion  RzSensePosition=on  RzSenseVelocity=on  RzSenseAcceleration=off  RzSenseTorqueForce=on  RzSenseLowerLimitTorqueForce=off  RzSenseUpperLimitTorqueForce=off
  HipForce : nesl_utility/PS-Simulink Converter  PhysicalDomain=network_engine_domain  SubClassName=ps_output  LeftPortType=input  RightPortType=output  PseudoPeriodic=off  Frequencies=[]  VectorFormat=1-D array  Unit=inherit  AffineConversion=off
  HipTorqueXInput : nesl_utility/PS-Simulink Converter  PhysicalDomain=network_engine_domain  SubClassName=ps_output  LeftPortType=input  RightPortType=output  PseudoPeriodic=off  Frequencies=[]  VectorFormat=1-D array  Unit=inherit  AffineConversion=off
  HipTorqueYInput : nesl_utility/PS-Simulink Converter  PhysicalDomain=network_engine_domain  SubClassName=ps_output  LeftPortType=input  RightPortType=output  PseudoPeriodic=off  Frequencies=[]  VectorFormat=1-D array  Unit=inherit  AffineConversion=off
  HipTorqueZInput : nesl_utility/PS-Simulink Converter  PhysicalDomain=network_engine_domain  SubClassName=ps_output  LeftPortType=input  RightPortType=output  PseudoPeriodic=off  Frequencies=[]  VectorFormat=1-D array  Unit=inherit  AffineConversion=off
  HipsAPX : nesl_utility/PS-Simulink Converter  PhysicalDomain=network_engine_domain  SubClassName=ps_output  LeftPortType=input  RightPortType=output  PseudoPeriodic=off  Frequencies=[]  VectorFormat=inherit  Unit=deg  AffineConversion=off
  HipsAPY : nesl_utility/PS-Simulink Converter  PhysicalDomain=network_engine_domain  SubClassName=ps_output  LeftPortType=input  RightPortType=output  PseudoPeriodic=off  Frequencies=[]  VectorFormat=inherit  Unit=deg  AffineConversion=off
  HipsAPZ : nesl_utility/PS-Simulink Converter  PhysicalDomain=network_engine_domain  SubClassName=ps_output  LeftPortType=input  RightPortType=output  PseudoPeriodic=off  Frequencies=[]  VectorFormat=inherit  Unit=deg  AffineConversion=off
  HipsAVX : nesl_utility/PS-Simulink Converter  PhysicalDomain=network_engine_domain  SubClassName=ps_output  LeftPortType=input  RightPortType=output  PseudoPeriodic=off  Frequencies=[]  VectorFormat=inherit  Unit=deg/s  AffineConversion=off
  HipsAVY : nesl_utility/PS-Simulink Converter  PhysicalDomain=network_engine_domain  SubClassName=ps_output  LeftPortType=input  RightPortType=output  PseudoPeriodic=off  Frequencies=[]  VectorFormat=inherit  Unit=deg/s  AffineConversion=off
  HipsAVZ : nesl_utility/PS-Simulink Converter  PhysicalDomain=network_engine_domain  SubClassName=ps_output  LeftPortType=input  RightPortType=output  PseudoPeriodic=off  Frequencies=[]  VectorFormat=inherit  Unit=deg/s  AffineConversion=off
  Simulink-PS Converter16 : nesl_utility/Simulink-PS Converter  PhysicalDomain=network_engine_domain  SubClassName=ps_input  LeftPortType=input  RightPortType=output  PseudoPeriodic=off  Frequencies=[]  NoiseDistribution=none  NoiseParameters=[]  Unit=deg  AffineConversion=off  FilteringAndDerivatives=provide  SimscapeFilterOrder=1  InputFilterTimeConstant=0.001  UdotUserProvided=2
  Simulink-PS Converter17 : nesl_utility/Simulink-PS Converter  PhysicalDomain=network_engine_domain  SubClassName=ps_input  LeftPortType=input  RightPortType=output  PseudoPeriodic=off  Frequencies=[]  NoiseDistribution=none  NoiseParameters=[]  Unit=deg  AffineConversion=off  FilteringAndDerivatives=provide  SimscapeFilterOrder=1  InputFilterTimeConstant=0.001  UdotUserProvided=2
  Simulink-PS Converter18 : nesl_utility/Simulink-PS Converter  PhysicalDomain=network_engine_domain  SubClassName=ps_input  LeftPortType=input  RightPortType=output  PseudoPeriodic=off  Frequencies=[]  NoiseDistribution=none  NoiseParameters=[]  Unit=deg  AffineConversion=off  FilteringAndDerivatives=provide  SimscapeFilterOrder=1  InputFilterTimeConstant=0.001  UdotUserProvided=2
  Simulink-PS Converter19 : nesl_utility/Simulink-PS Converter  PhysicalDomain=network_engine_domain  SubClassName=ps_input  LeftPortType=input  RightPortType=output  PseudoPeriodic=off  Frequencies=[]  NoiseDistribution=none  NoiseParameters=[]  Unit=m  AffineConversion=off  FilteringAndDerivatives=provide  SimscapeFilterOrder=1  InputFilterTimeConstant=0.001  UdotUserProvided=2
  Simulink-PS Converter20 : nesl_utility/Simulink-PS Converter  PhysicalDomain=network_engine_domain  SubClassName=ps_input  LeftPortType=input  RightPortType=output  PseudoPeriodic=off  Frequencies=[]  NoiseDistribution=none  NoiseParameters=[]  Unit=m  AffineConversion=off  FilteringAndDerivatives=provide  SimscapeFilterOrder=1  InputFilterTimeConstant=0.001  UdotUserProvided=2
  Simulink-PS Converter21 : nesl_utility/Simulink-PS Converter  PhysicalDomain=network_engine_domain  SubClassName=ps_input  LeftPortType=input  RightPortType=output  PseudoPeriodic=off  Frequencies=[]  NoiseDistribution=none  NoiseParameters=[]  Unit=m  AffineConversion=off  FilteringAndDerivatives=provide  SimscapeFilterOrder=1  InputFilterTimeConstant=0.001  UdotUserProvided=2
  TranslationForceXInput : nesl_utility/PS-Simulink Converter  PhysicalDomain=network_engine_domain  SubClassName=ps_output  LeftPortType=input  RightPortType=output  PseudoPeriodic=off  Frequencies=[]  VectorFormat=1-D array  Unit=inherit  AffineConversion=off
  TranslationForceYInput : nesl_utility/PS-Simulink Converter  PhysicalDomain=network_engine_domain  SubClassName=ps_output  LeftPortType=input  RightPortType=output  PseudoPeriodic=off  Frequencies=[]  VectorFormat=1-D array  Unit=inherit  AffineConversion=off
  TranslationForceZInput : nesl_utility/PS-Simulink Converter  PhysicalDomain=network_engine_domain  SubClassName=ps_output  LeftPortType=input  RightPortType=output  PseudoPeriodic=off  Frequencies=[]  VectorFormat=1-D array  Unit=inherit  AffineConversion=off
  Hips : PMIOPort  Side=Right
  Base : PMIOPort  Port=2  Side=Left
  tag scope: HipPositionX=global, HipPositionY=global, HipPositionZ=global, HipVelocityX=global, HipVelocityY=global, HipVelocityZ=global
  wires:
  [FcnOutHipAccelerationZ] -> Simulink-PS Converter18/3
  [FcnOutTranslationAccelerationZ] -> Simulink-PS Converter21/3
  [FcnOutHipAccelerationY] -> Simulink-PS Converter17/3
  [FcnOutTranslationPositionX] -> Simulink-PS Converter19/1
  [FcnOutTranslationPositionY] -> Simulink-PS Converter20/1
  [FcnOutHipVelocityZ] -> Simulink-PS Converter18/2
  [FcnOutHipPositionX] -> Simulink-PS Converter16/1
  [FcnOutHipAccelerationX] -> Simulink-PS Converter16/3
  [FcnOutTranslationVelocityX] -> Simulink-PS Converter19/2
  [FcnOutHipPositionY] -> Simulink-PS Converter17/1
  [FcnOutHipVelocityX] -> Simulink-PS Converter16/2
  [FcnOutTranslationAccelerationX] -> Simulink-PS Converter19/3
  [FcnOutTranslationPositionZ] -> Simulink-PS Converter21/1
  [FcnOutTranslationVelocityY] -> Simulink-PS Converter20/2
  [FcnOutHipVelocityY] -> Simulink-PS Converter17/2
  [FcnOutTranslationVelocityZ] -> Simulink-PS Converter21/2
  [FcnOutHipPositionZ] -> Simulink-PS Converter18/1
  [FcnOutTranslationAccelerationY] -> Simulink-PS Converter20/3
  HipsAVZ/1 -> [HipVelocityZ]  "HipVelocityZ"
  HipsAPX/1 -> [HipPositionX]  "HipPositionX"
  HipsAPY/1 -> [HipPositionY]  "HipPositionY"
  HipsAVX/1 -> [HipVelocityX]  "HipVelocityX"
  HipsAPZ/1 -> [HipPositionZ]  "HipPositionZ"
  HipsAVY/1 -> [HipVelocityY]  "HipVelocityY"
  BaseonHipTorqueLocalBaseRefFrame/1 -> BaseonHipTorqueGlobalPseudoGRT/2  "HipTorqueLocal"
  HipForce/1 -> BaseonHipForceGlobalPseudoGRF/2  "BaseonHipForceLocalBaseRefFrame"
  [RVectorHipJointBasetoGlobal] -> BaseonHipForceGlobalPseudoGRF/1, BaseonHipTorqueGlobalPseudoGRT/1
  HipTorqueXInput/1 -> ?  "HipTorqueXInput"
  TranslationForceZInput/1 -> ?  "TranslationForceZInput"
  TranslationForceYInput/1 -> ?  "TranslationForceYInput"
  TranslationForceXInput/1 -> ?  "TranslationForceXInput"
  HipTorqueYInput/1 -> ?  "HipTorqueYInput"
  HipTorqueZInput/1 -> ?  "HipTorqueZInput"
  connections:
  Simulink-PS Converter21/RConn1 -- Hip Joint1/LConn4
  Simulink-PS Converter18/RConn1 -- Hip Joint1/LConn7
  Simulink-PS Converter17/RConn1 -- Hip Joint1/LConn6
  Simulink-PS Converter16/RConn1 -- Hip Joint1/LConn5
  Simulink-PS Converter19/RConn1 -- Hip Joint1/LConn2
  Simulink-PS Converter20/RConn1 -- Hip Joint1/LConn3
  Base/RConn1 -- Hip Joint1/LConn1
  Hips/RConn1 -- Hip Joint1/RConn1
  HipsAPX/LConn1 -- Hip Joint1/RConn5
  HipsAVX/LConn1 -- Hip Joint1/RConn6
  HipsAPY/LConn1 -- Hip Joint1/RConn8
  HipsAVY/LConn1 -- Hip Joint1/RConn9
  HipsAPZ/LConn1 -- Hip Joint1/RConn11
  HipsAVZ/LConn1 -- Hip Joint1/RConn12
  HipForce/LConn1 -- Hip Joint1/RConn14
  TranslationForceXInput/LConn1 -- Hip Joint1/RConn2
  TranslationForceYInput/LConn1 -- Hip Joint1/RConn3
  TranslationForceZInput/LConn1 -- Hip Joint1/RConn4
  HipTorqueXInput/LConn1 -- Hip Joint1/RConn7
  HipTorqueYInput/LConn1 -- Hip Joint1/RConn10
  HipTorqueZInput/LConn1 -- Hip Joint1/RConn13
  BaseonHipTorqueLocalBaseRefFrame/LConn1 -- Hip Joint1/RConn15
